simulink model "high_level"  (Simulink 8.3)
settings: Solver=ode45  StartTime=0.0  StopTime=24/3000  RelTol=1e-6
PreLoadFcn:
  | load one_stage.mat
libraries: simulink_extras x2, simulink x2, dspmlti4 x1
(part 1 of 2)
settings Model: Creator=abehbood  LastModifiedBy=KRISH
settings SolverCC: ConsecutiveZCsStepRelTol=128*eps  ZeroCrossControl=DisableAll
settings DataIOCC: LimitDataPoints=off  SaveFormat=StructureWithTime
settings OptimizationCC: ExpressionDepthLimit=2147483647  InitFltsAndDblsToZero=on
settings DebuggingCC: SaveWithParameterizedLinksMsg=none  SignalResolutionControl=TryResolveAllWithWarning  FcnCallInpInsideContextMsg=UseLocalSettings  StrictBusMsg=Warning
settings SFSimCC: SimParseCustomCode=off
settings GRTTargetCC: TargetFcnLib=ansi_tfl_tmw.mat
settings ConfigurationSet: Description=SimMechanics 2G

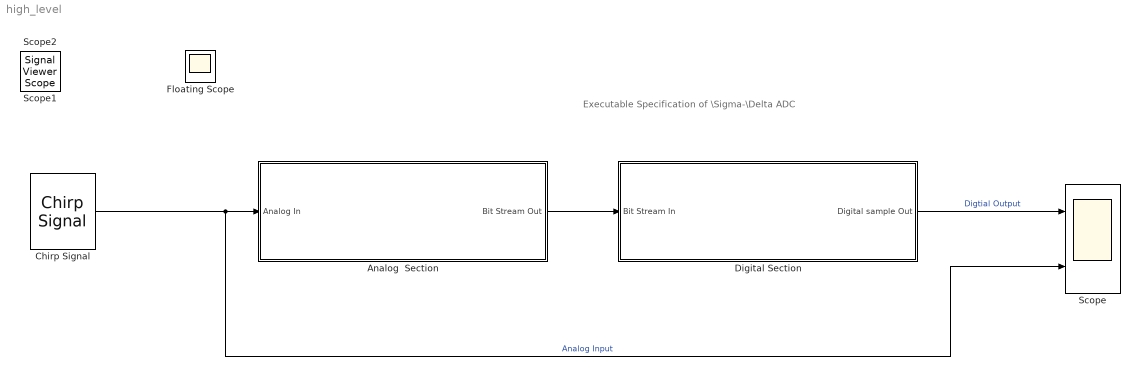
== system high_level ==
  note: Executable Specification of
      | \Sigma-\Delta ADC
  Analog  Section : Subsystem
  Chirp Signal : simulink/Sources/Chirp Signal  f1=.1  T=6/3000  f2=1000
  Digital Section : Subsystem
  Scope : Scope  NumInputPorts=2
      settings: TimeRange=0.008  YMin=-1~-1  YMax=1~1
  Floating Scope : Scope
      settings: Floating=on  YMin=-1  YMax=1
  Scope1 : SignalViewerScope  IOType=viewer  RefreshTime=0.035000
  Scope2 : SignalViewerScope  IOType=viewer  RefreshTime=0.035000
  wires:
  Analog  Section/1(Bit Stream Out) -> Digital Section/1(Bit Stream In)
  Digital Section/1(Digital sample Out) -> Scope/1  "Digtial Output"
  Chirp Signal/1 -> Scope/2, Analog  Section/1(Analog In)  "Analog Input"

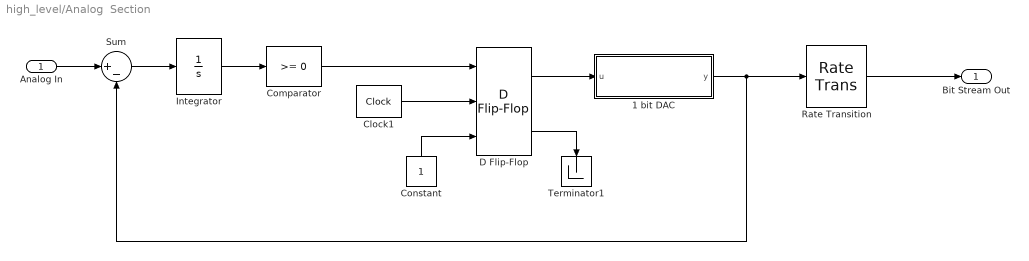
== system high_level/Analog  Section ==
  Analog In : Inport
  1 bit DAC : MATLAB Function  TreatAsAtomicUnit=on
  Clock1 : simulink_extras/Flip Flops/Clock  SystemSampleTime=-1  MaskParam1=1/(48e3*64)
  Comparator : simulink/Logic and Bit Operations/Compare To Zero  SystemSampleTime=-1  relop=>=  LogicOutDataTypeMode=boolean  ZeroCross=off
  Constant : Constant  SampleTime=0
  D Flip-Flop : simulink_extras/Flip Flops/D Flip-Flop  SystemSampleTime=-1
  Integrator : Integrator
  Rate Transition : RateTransition  OutPortSampleTime=1/(48e3*64)
  Sum : Sum  Inputs=|+-
  Terminator1 : Terminator
  Bit Stream Out : Outport  OutDataTypeStr=double
  wires:
  Sum/1 -> Integrator/1
  Integrator/1 -> Comparator/1
  Comparator/1 -> D Flip-Flop/1
  Analog In/1 -> Sum/1
  D Flip-Flop/2 -> Terminator1/1
  Clock1/1 -> D Flip-Flop/2
  D Flip-Flop/1 -> 1 bit DAC/1(u)
  Constant/1 -> D Flip-Flop/3
  1 bit DAC/1(y) -> Sum/2, Rate Transition/1
  Rate Transition/1 -> Bit Stream Out/1
